simulink model "comparando_modelos"  (R2012b)
settings: Solver=VariableStepDiscrete  StartTime=0.0  StopTime=15  MaxStep=Ts  RelTol=1e-3
undefined symbols (not defined in the file): DiscIntNeverNeededParam, Ts
libraries: simulink x6, slident x4
settings Model: Creator=Elisa  LastModifiedBy=Carlos

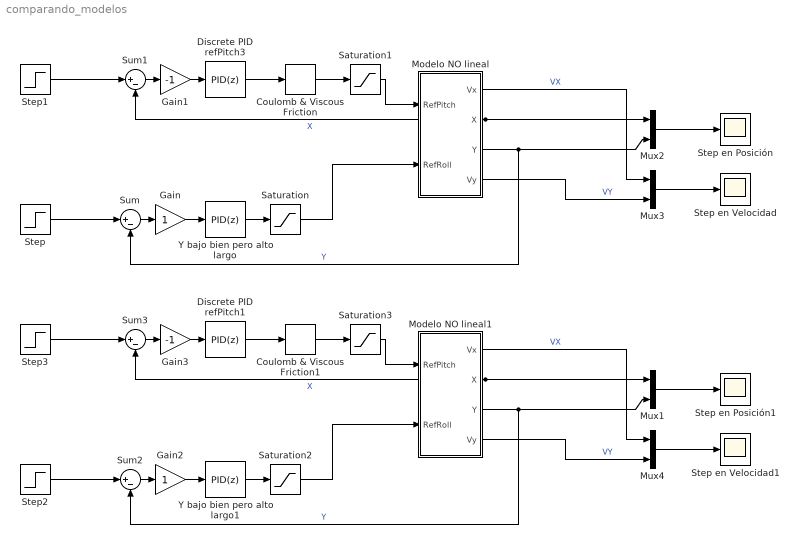
== system comparando_modelos ==
  " Modelo NO lineal" : Subsystem
  " Modelo NO lineal1" : Subsystem
  Coulomb & Viscous Friction : simulink/Discontinuities/Coulomb & Viscous Friction  offset=0.04  gain=1
  Coulomb & Viscous Friction1 : simulink/Discontinuities/Coulomb & Viscous Friction  offset=0.04  gain=1
  Discrete PID refPitch1 : simulink/Continuous/PID Controller  Controller=PID  TimeDomain=Discrete-time  SampleTime=Ts  IntegratorMethod=Forward Euler  FilterMethod=Forward Euler  Form=Parallel  P=0.1  I=0  D=0.05  N=12  InitialConditionSource=internal  InitialConditionForIntegrator=0  InitialConditionForFilter=0  ExternalReset=none  LimitOutput=off  UpperSaturationLimit=inf  LowerSaturationLimit=-inf  LinearizeAsGain=off  AntiWindupMode=none  Kb=1  TrackingMode=off  Kt=1  PParamMin=[]  PParamMax=[]  IParamMin=[]  IParamMax=[]  DParamMin=[]  DParamMax=[]  NParamMin=[]  NParamMax=[]  KbParamMin=[]  KbParamMax=[]  KtParamMin=[]  KtParamMax=[]  POutMin=[]  POutMax=[]  IOutMin=[]  IOutMax=[]  DOutMin=[]  DOutMax=[]  NOutMin=[]  NOutMax=[]  KbOutMin=[]  KbOutMax=[]  KtOutMin=[]  KtOutMax=[]  IntegratorOutMin=[]  IntegratorOutMax=[]  FilterOutMin=[]  FilterOutMax=[]  SumOutMin=[]  SumOutMax=[]  SumI1OutMin=[]  SumI1OutMax=[]  SumI2OutMin=[]  SumI2OutMax=[]  SumI3OutMin=[]  SumI3OutMax=[]  SumDOutMin=[]  SumDOutMax=[]  SaturationOutMin=[]  SaturationOutMax=[]  IntegratorContinuousStateAttributes=''  IntegratorStateMustResolveToSignalObject=off  IntegratorRTWStateStorageClass=Auto  FilterContinuousStateAttributes=''  FilterStateMustResolveToSignalObject=off  FilterRTWStateStorageClass=Auto
  Discrete PID refPitch3 : simulink/Continuous/PID Controller  Controller=PID  TimeDomain=Discrete-time  SampleTime=Ts  IntegratorMethod=Forward Euler  FilterMethod=Forward Euler  Form=Parallel  P=0.1  I=0  D=0.05  N=12  InitialConditionSource=internal  InitialConditionForIntegrator=0  InitialConditionForFilter=0  ExternalReset=none  LimitOutput=off  UpperSaturationLimit=inf  LowerSaturationLimit=-inf  LinearizeAsGain=off  AntiWindupMode=none  Kb=1  TrackingMode=off  Kt=1  PParamMin=[]  PParamMax=[]  IParamMin=[]  IParamMax=[]  DParamMin=[]  DParamMax=[]  NParamMin=[]  NParamMax=[]  KbParamMin=[]  KbParamMax=[]  KtParamMin=[]  KtParamMax=[]  POutMin=[]  POutMax=[]  IOutMin=[]  IOutMax=[]  DOutMin=[]  DOutMax=[]  NOutMin=[]  NOutMax=[]  KbOutMin=[]  KbOutMax=[]  KtOutMin=[]  KtOutMax=[]  IntegratorOutMin=[]  IntegratorOutMax=[]  FilterOutMin=[]  FilterOutMax=[]  SumOutMin=[]  SumOutMax=[]  SumI1OutMin=[]  SumI1OutMax=[]  SumI2OutMin=[]  SumI2OutMax=[]  SumI3OutMin=[]  SumI3OutMax=[]  SumDOutMin=[]  SumDOutMax=[]  SaturationOutMin=[]  SaturationOutMax=[]  IntegratorContinuousStateAttributes=''  IntegratorStateMustResolveToSignalObject=off  IntegratorRTWStateStorageClass=Auto  FilterContinuousStateAttributes=''  FilterStateMustResolveToSignalObject=off  FilterRTWStateStorageClass=Auto
  Gain : Gain
  Gain1 : Gain  Gain=-1  SampleTime=Ts
  Gain2 : Gain
  Gain3 : Gain  Gain=-1  SampleTime=Ts
  Mux{1..4} (4 alike) : Mux  Inputs=2
  Saturation{,1..3} (4 alike) : Saturate  UpperLimit=1  LowerLimit=-1  SampleTime=Ts
  Step{,1..3} (4 alike) : Step  Time=0.06  After=10  SampleTime=Ts
  Step en Posición : Scope
      settings: ShowLegends=on  TimeRange=15  YMin=9.640410958904109  YMax=10  SaveName=PIDtestscdata  SampleInput=on  SampleTime=Ts
  Step en Posición1 : Scope
      settings: ShowLegends=on  SaveName=PIDtestscdata1  SampleInput=on  SampleTime=Ts
  Step en Velocidad : Scope
      settings: ShowLegends=on  SampleInput=on  SampleTime=Ts
  Step en Velocidad1 : Scope
      settings: ShowLegends=on  SampleInput=on  SampleTime=Ts
  Sum{,1..3} (4 alike) : Sum  Inputs=|+-
  Y bajo bien pero alto largo : simulink/Continuous/PID Controller  Controller=PID  TimeDomain=Discrete-time  SampleTime=Ts  IntegratorMethod=Forward Euler  FilterMethod=Forward Euler  Form=Parallel  P=1.5  I=0  D=0.9  N=27  InitialConditionSource=internal  InitialConditionForIntegrator=0  InitialConditionForFilter=0  ExternalReset=none  LimitOutput=off  UpperSaturationLimit=inf  LowerSaturationLimit=-inf  LinearizeAsGain=off  AntiWindupMode=none  Kb=1  TrackingMode=off  Kt=1  PParamMin=[]  PParamMax=[]  IParamMin=[]  IParamMax=[]  DParamMin=[]  DParamMax=[]  NParamMin=[]  NParamMax=[]  KbParamMin=[]  KbParamMax=[]  KtParamMin=[]  KtParamMax=[]  POutMin=[]  POutMax=[]  IOutMin=[]  IOutMax=[]  DOutMin=[]  DOutMax=[]  NOutMin=[]  NOutMax=[]  KbOutMin=[]  KbOutMax=[]  KtOutMin=[]  KtOutMax=[]  IntegratorOutMin=[]  IntegratorOutMax=[]  FilterOutMin=[]  FilterOutMax=[]  SumOutMin=[]  SumOutMax=[]  SumI1OutMin=[]  SumI1OutMax=[]  SumI2OutMin=[]  SumI2OutMax=[]  SumI3OutMin=[]  SumI3OutMax=[]  SumDOutMin=[]  SumDOutMax=[]  SaturationOutMin=[]  SaturationOutMax=[]  IntegratorContinuousStateAttributes=''  IntegratorStateMustResolveToSignalObject=off  IntegratorRTWStateStorageClass=Auto  FilterContinuousStateAttributes=''  FilterStateMustResolveToSignalObject=off  FilterRTWStateStorageClass=Auto
  Y bajo bien pero alto largo1 : simulink/Continuous/PID Controller  Controller=PID  TimeDomain=Discrete-time  SampleTime=Ts  IntegratorMethod=Forward Euler  FilterMethod=Forward Euler  Form=Parallel  P=1.5  I=0  D=1  N=27  InitialConditionSource=internal  InitialConditionForIntegrator=0  InitialConditionForFilter=0  ExternalReset=none  LimitOutput=off  UpperSaturationLimit=inf  LowerSaturationLimit=-inf  LinearizeAsGain=off  AntiWindupMode=none  Kb=1  TrackingMode=off  Kt=1  PParamMin=[]  PParamMax=[]  IParamMin=[]  IParamMax=[]  DParamMin=[]  DParamMax=[]  NParamMin=[]  NParamMax=[]  KbParamMin=[]  KbParamMax=[]  KtParamMin=[]  KtParamMax=[]  POutMin=[]  POutMax=[]  IOutMin=[]  IOutMax=[]  DOutMin=[]  DOutMax=[]  NOutMin=[]  NOutMax=[]  KbOutMin=[]  KbOutMax=[]  KtOutMin=[]  KtOutMax=[]  IntegratorOutMin=[]  IntegratorOutMax=[]  FilterOutMin=[]  FilterOutMax=[]  SumOutMin=[]  SumOutMax=[]  SumI1OutMin=[]  SumI1OutMax=[]  SumI2OutMin=[]  SumI2OutMax=[]  SumI3OutMin=[]  SumI3OutMax=[]  SumDOutMin=[]  SumDOutMax=[]  SaturationOutMin=[]  SaturationOutMax=[]  IntegratorContinuousStateAttributes=''  IntegratorStateMustResolveToSignalObject=off  IntegratorRTWStateStorageClass=Auto  FilterContinuousStateAttributes=''  FilterStateMustResolveToSignalObject=off  FilterRTWStateStorageClass=Auto
  wires:
  Step1/1 -> Sum1/1
  Y bajo bien pero alto largo/1 -> Saturation/1
  Sum/1 -> Gain/1
  Gain/1 -> Y bajo bien pero alto largo/1
  Sum1/1 -> Gain1/1
  Gain1/1 -> Discrete PID refPitch3/1
  Discrete PID refPitch3/1 -> Coulomb & Viscous Friction/1
  Mux3/1 -> Step en Velocidad/1
  Mux2/1 -> Step en Posición/1
  Step/1 -> Sum/1
  " Modelo NO lineal"/1(Vx) -> Mux3/1  "VX"
  " Modelo NO lineal"/2(X) -> Mux2/1, Sum1/2  "X"
  " Modelo NO lineal"/3(Y) -> Sum/2, Mux2/2  "Y"
  " Modelo NO lineal"/4(Vy) -> Mux3/2  "VY"
  Saturation/1 -> " Modelo NO lineal"/2(RefRoll)
  Saturation1/1 -> " Modelo NO lineal"/1(RefPitch)
  Coulomb & Viscous Friction/1 -> Saturation1/1
  Step3/1 -> Sum3/1
  Y bajo bien pero alto largo1/1 -> Saturation2/1
  Sum2/1 -> Gain2/1
  Gain2/1 -> Y bajo bien pero alto largo1/1
  Sum3/1 -> Gain3/1
  Gain3/1 -> Discrete PID refPitch1/1
  Discrete PID refPitch1/1 -> Coulomb & Viscous Friction1/1
  Mux4/1 -> Step en Velocidad1/1
  Mux1/1 -> Step en Posición1/1
  Step2/1 -> Sum2/1
  " Modelo NO lineal1"/1(Vx) -> Mux4/1  "VX"
  " Modelo NO lineal1"/2(X) -> Mux1/1, Sum3/2  "X"
  " Modelo NO lineal1"/3(Y) -> Sum2/2, Mux1/2  "Y"
  " Modelo NO lineal1"/4(Vy) -> Mux4/2  "VY"
  Saturation2/1 -> " Modelo NO lineal1"/2(RefRoll)
  Saturation3/1 -> " Modelo NO lineal1"/1(RefPitch)
  Coulomb & Viscous Friction1/1 -> Saturation3/1

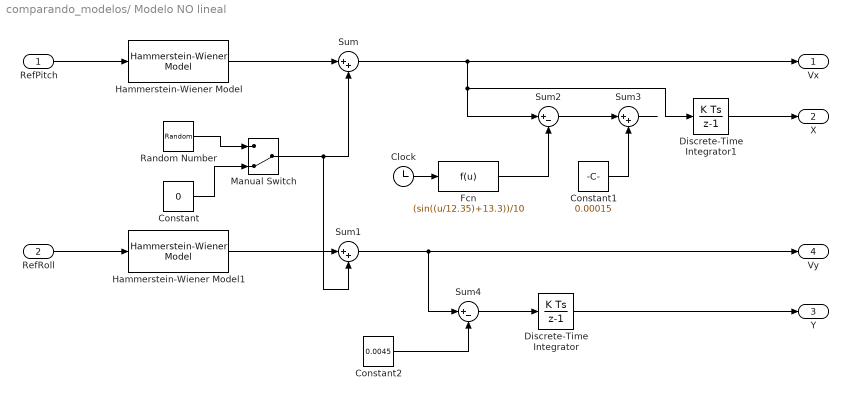
== system comparando_modelos/ Modelo NO lineal ==
  RefPitch : Inport  PortDimensions=1  SampleTime=0.06
  RefRoll : Inport  Port=2  PortDimensions=1  SampleTime=0.06
  Clock : Clock
      settings: Decimation=2
  Constant : Constant  Value=0  SampleTime=Ts
  Constant1 : Constant  Value=0.00015
  Constant2 : Constant  Value=0.0045
  Discrete-Time Integrator : DiscreteIntegrator  gainval=1  SampleTime=Ts  ICPrevOutput=DiscIntNeverNeededParam  ICPrevScaledInput=DiscIntNeverNeededParam
  Discrete-Time Integrator1 : DiscreteIntegrator  SampleTime=Ts  ICPrevOutput=DiscIntNeverNeededParam  ICPrevScaledInput=DiscIntNeverNeededParam
  Fcn : Fcn  Expr=(sin((u/12.35)+13.3))/10  SampleTime=Ts
  Hammerstein-Wiener Model : slident/Hammerstein-Wiener Model  sys=vx123_nlhw113_pic2  IC=Zero  X0i=0
  Hammerstein-Wiener Model1 : slident/Hammerstein-Wiener Model  sys=vy123_nlhw111  IC=Zero  X0i=0
  Manual Switch : ManualSwitch  CurrentSetting=0
  Random Number : RandomNumber  Variance=0.3  SampleTime=Ts
  Sum : Sum  Inputs=|++
  Sum1 : Sum  Inputs=|++
  Sum2 : Sum  Inputs=|+-
  Sum3 : Sum  Inputs=|++
  Sum4 : Sum  Inputs=|+-
  Vx : Outport
  X : Outport  Port=2
  Y : Outport  Port=3
  Vy : Outport  Port=4
  wires:
  Hammerstein-Wiener Model/1 -> Sum/1
  RefRoll/1 -> Hammerstein-Wiener Model1/1
  RefPitch/1 -> Hammerstein-Wiener Model/1
  Discrete-Time Integrator/1 -> Y/1
  Discrete-Time Integrator1/1 -> X/1
  Hammerstein-Wiener Model1/1 -> Sum1/1
  Random Number/1 -> Manual Switch/1
  Constant/1 -> Manual Switch/2
  Manual Switch/1 -> Sum/2, Sum1/2
  Sum/1 -> Discrete-Time Integrator1/1, Sum2/1, Vx/1
  Sum2/1 -> Sum3/1
  Sum3/1 -> ?
  Constant1/1 -> Sum3/2
  Fcn/1 -> Sum2/2
  Clock/1 -> Fcn/1
  Sum1/1 -> Sum4/1, Vy/1
  Constant2/1 -> Sum4/2
  Sum4/1 -> Discrete-Time Integrator/1

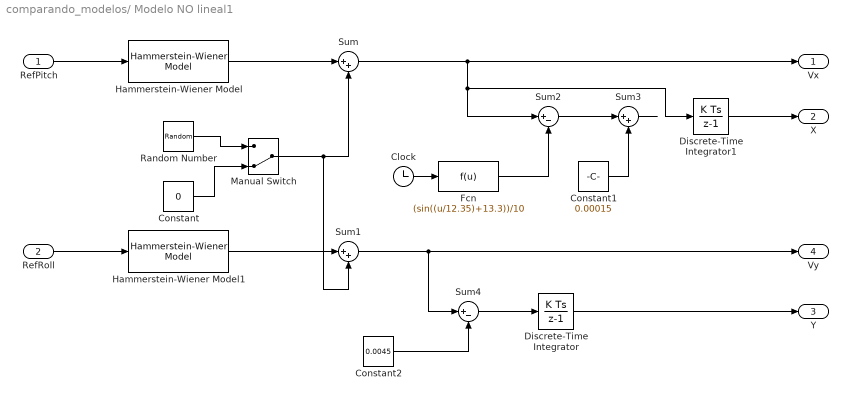
== system comparando_modelos/ Modelo NO lineal1 ==
  RefPitch : Inport  PortDimensions=1  SampleTime=0.06
  RefRoll : Inport  Port=2  PortDimensions=1  SampleTime=0.06
  Clock : Clock
      settings: Decimation=2
  Constant : Constant  Value=0  SampleTime=Ts
  Constant1 : Constant  Value=0.00015
  Constant2 : Constant  Value=0.0045
  Discrete-Time Integrator : DiscreteIntegrator  gainval=1  SampleTime=Ts  ICPrevOutput=DiscIntNeverNeededParam  ICPrevScaledInput=DiscIntNeverNeededParam
  Discrete-Time Integrator1 : DiscreteIntegrator  SampleTime=Ts  ICPrevOutput=DiscIntNeverNeededParam  ICPrevScaledInput=DiscIntNeverNeededParam
  Fcn : Fcn  Expr=(sin((u/12.35)+13.3))/10  SampleTime=Ts
  Hammerstein-Wiener Model : slident/Hammerstein-Wiener Model  sys=vx123_nlhw113_pic2  IC=Zero  X0i=0
  Hammerstein-Wiener Model1 : slident/Hammerstein-Wiener Model  sys=vy123_nlhw111  IC=Zero  X0i=0
  Manual Switch : ManualSwitch  CurrentSetting=0
  Random Number : RandomNumber  Variance=0.3  SampleTime=Ts
  Sum : Sum  Inputs=|++
  Sum1 : Sum  Inputs=|++
  Sum2 : Sum  Inputs=|+-
  Sum3 : Sum  Inputs=|++
  Sum4 : Sum  Inputs=|+-
  Vx : Outport
  X : Outport  Port=2
  Y : Outport  Port=3
  Vy : Outport  Port=4
  wires:
  Hammerstein-Wiener Model/1 -> Sum/1
  RefRoll/1 -> Hammerstein-Wiener Model1/1
  RefPitch/1 -> Hammerstein-Wiener Model/1
  Discrete-Time Integrator/1 -> Y/1
  Discrete-Time Integrator1/1 -> X/1
  Hammerstein-Wiener Model1/1 -> Sum1/1
  Random Number/1 -> Manual Switch/1
  Constant/1 -> Manual Switch/2
  Manual Switch/1 -> Sum/2, Sum1/2
  Sum/1 -> Discrete-Time Integrator1/1, Sum2/1, Vx/1
  Sum2/1 -> Sum3/1
  Sum3/1 -> ?
  Constant1/1 -> Sum3/2
  Fcn/1 -> Sum2/2
  Clock/1 -> Fcn/1
  Sum1/1 -> Sum4/1, Vy/1
  Constant2/1 -> Sum4/2
  Sum4/1 -> Discrete-Time Integrator/1
